simulink model "MomentForceCBAgent"  (Simulink 7.1)
settings: Solver=ode45  SolverMode=SingleTasking  StartTime=0.0  StopTime=10.0  RelTol=1e-3  AbsTol=1e-6
settings Model: Creator=The MathWorks Inc.  LastModifiedBy=suarezjl  ExtModeTrigMode=oneshot  ExtModeArmWhenConnect=off  ExtModeAutoUpdateStatusClock=off
settings DataIOCC: LimitDataPoints=off  SignalLoggingName=logsOut
settings OptimizationCC: BooleanDataType=off  InlineInvariantSignals=on
settings DebuggingCC: SaveWithParameterizedLinksMsg=none  CheckExecutionContextPreStartOutputMsg=on  CheckExecutionContextRuntimeOutputMsg=on  SignalResolutionControl=TryResolveAllWithWarning  SolverPrmCheckMsg=none  MultiTaskDSMMsg=warning  MultiTaskCondExecSysMsg=none  IntegerOverflowMsg=none  StrictBusMsg=None
settings HardwareCC: TargetUnknown=on
settings ModelReferenceCC: UpdateModelReferenceTargets=IfOutOfDate
settings RTWCC: IncludeERTFirstTime=on
settings GRTTargetCC: TargetFcnLib=ansi_tfl_tmw.mat

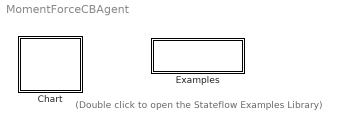
== system MomentForceCBAgent ==
  note: (Double click to open the
      | Stateflow Examples Library)
  Chart : Stateflow chart
  Examples : Subsystem
      settings: OpenFcn=sf('Private','sf_examples')
      mask Display: disp('Examples')

== system MomentForceCBAgent/Examples ==

== stateflow chart Chart ==
  state Initialize
    \\Octavia\ISACControlBasisModule\MomentForceCB\MomentForceCBLeft.Initialize()
    \\Octavia\ISACControlBasisModule\MomentForceCB\MomentForceCBRight.Initialize()
    \\Octavia\ISACControlBasisModule\RightModule\Arm\ArmController.DoHomingRoutine()
    \\Octavia\ISACControlBasisModule\MomentForceCB\StateMachine.Wait(5000)
    \\Octavia\ISACControlBasisModule\LeftModule\Arm\ArmController.DoHomingRoutine()
    \\Octavia\ISACControlBasisModule\MomentForceCB\StateMachine.Wait(5000)
  state ControlBasis
    \\Octavia\ISACControlBasisModule\RightModule\Arm\ArmController.Move()
    \\Octavia\ISACControlBasisModule\LeftModule\Arm\ArmController.Move()
    \\Octavia\ISACControlBasisModule\MomentForceCB\MomentForceCBLeft.ComputeControlBasis()
    \\Octavia\ISACControlBasisModule\MomentForceCB\MomentForceCBRight.ComputeControlBasis()
  state End
    \\Octavia\ISACControlBasisModule\MomentForceCB\MomentForceCBLeft.Close()
    \\Octavia\ISACControlBasisModule\MomentForceCB\MomentForceCBRight.Close()
    \\Octavia\ISACControlBasisModule\RightModule\ForceSensor\StateMachine.Stop()
    \\Octavia\ISACControlBasisModule\LeftModule\ForceSensor\StateMachine.Stop()
    \\Octavia\ISACControlBasisModule\VirtualContact\StateMachine.Stop()
  state StartStateMachines
    \\Octavia\ISACControlBasisModule\RightModule\ForceSensor\StateMachine.LoadSM()
    \\Octavia\ISACControlBasisModule\LeftModule\ForceSensor\StateMachine.LoadSM()
    \\Octavia\ISACControlBasisModule\VirtualContact\StateMachine.LoadSM()
    \\Octavia\ISACControlBasisModule\RightModule\ForceSensor\StateMachine.Start()
    \\Octavia\ISACControlBasisModule\LeftModule\ForceSensor\StateMachine.Start()
    \\Octavia\ISACControlBasisModule\VirtualContact\StateMachine.Start()
    \\Octavia\ISACControlBasisModule\MomentForceCB\StateMachine.Wait(2500)
    \\Octavia\ISACControlBasisModule\RightModule\ForceSensor\ATISensor.BiasSensor()
    \\Octavia\ISACControlBasisModule\LeftModule\ForceSensor\ATISensor.BiasSensor()
  (default) -> Initialize : Start
  Initialize -> StartStateMachines : Signal="Next"
  ControlBasis -> ControlBasis [order 1] : Default
  ControlBasis -> End [order 2] : Signal="Next"
  StartStateMachines -> ControlBasis : Signal="Next"
